simulink model "Motoring_Gear"  (R2024a)
settings: Solver=VariableStepAuto  StartTime=0.0  StopTime=2  FixedStep=1e-6  MaxStep=1e-6  RelTol=1e-6
values from neighbouring files (symbols this model uses):
  B_mod = 0    [Motoring_Gear_param.m]
  Bdc = 1e-4    (= 0.0001)    [Motoring_Gear_param.m]
  BL = 5    [Motoring_Gear_param.m]
  Bs = 1e10    (= 10000000000)    [Motoring_Gear_param.m]
  Bsn = 0    [Motoring_Gear_param.m]
  flux = 0.0563    [Motoring_Gear_param.m]
  J_mod = 5.71e-4    (= 0.000571)    [Motoring_Gear_param.m]
  Jdc = 0.0003    [Motoring_Gear_param.m]
  Jsn = 3.16e-4    (= 0.000316)    [Motoring_Gear_param.m]
  Kag = 0.001    [Motoring_Gear_param.m]
  Kc = 1000000    [Motoring_Gear_param.m]
  Ke = 0.0164    [Motoring_Gear_param.m]
  Kt = 0.0164    [Motoring_Gear_param.m]
  Ld = 3e-5    (= 3e-05)    [Motoring_Gear_param.m]
  Ldc = 8.76e-5    (= 8.76e-05)    [Motoring_Gear_param.m]
  Lq = 3e-5    (= 3e-05)    [Motoring_Gear_param.m]
  Pa = 2    [Motoring_Gear_param.m]
  Psn = 9    [Motoring_Gear_param.m]
  q_mod = 11    [Motoring_Gear_param.m]
  Rs = 0.01    [Motoring_Gear_param.m]
  Rs_dc = 0.01    [Motoring_Gear_param.m]
  velocity_Ki_pi = Bdc*motor_bw    (= 0.0628318530718)    [Motoring_Gear_param.m]
  velocity_Kp_pi = Jdc*motor_bw    (= 0.188495559215)    [Motoring_Gear_param.m]
libraries: cstblocks x2
(part 2 of 2)

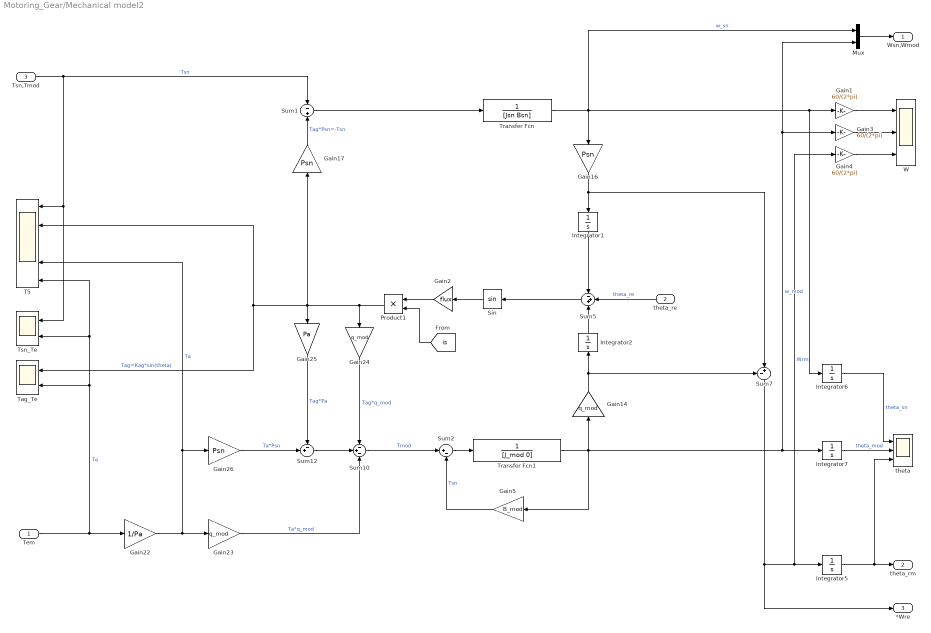
== system Motoring_Gear/Mechanical model2 ==
  Tem : Inport
  theta_re : Inport  Port=2
  Tsn,Tmod : Inport  Port=3
  Gain1 : Gain  Gain=60/(2*pi)
  Gain14 : Gain  Gain=q_mod
  Gain16 : Gain  Gain=Psn
  Gain17 : Gain  Gain=Psn
  Gain2 : Gain  Gain=flux
  Gain22 : Gain  Gain=1/Pa
  Gain23 : Gain  Gain=q_mod
  Gain24 : Gain  Gain=q_mod
  Gain25 : Gain  Gain=Pa
  Gain26 : Gain  Gain=Psn
  Gain3 : Gain  Gain=60/(2*pi)
  Gain4 : Gain  Gain=60/(2*pi)
  Gain5 : Gain  Gain=B_mod
  Integrator{1..2,5..7} (5 alike) : Integrator
  Mux : Mux  Inputs=2
  Product1 : Product
  Sin : Trigonometry
  Sum1 : Sum  Inputs=-|+
  Sum10 : Sum  Inputs=-+-
  Sum12 : Sum  Inputs=-+|
  Sum2 : Sum  Inputs=|+-
  Sum5 : Sum  Inputs=-++
  Sum7 : Sum  Inputs=-+|
  T5 : Scope  NumInputPorts=5
  Tag_Te : Scope  NumInputPorts=2
  Transfer Fcn : TransferFcn  Denominator=[Jsn Bsn]
  Transfer Fcn1 : TransferFcn  Denominator=[J_mod 0]
  Tsn_Te : Scope  NumInputPorts=2
  W : Scope  NumInputPorts=3
  theta : Scope  NumInputPorts=3
  Wsn,Wmod : Outport
  theta_rm : Outport  Port=2
  *Wre : Outport  Port=3
  wires:
  Gain4/1 -> W/3
  Gain3/1 -> W/2
  Gain1/1 -> W/1
  Tsn,Tmod/1 -> Sum1/1, Tsn_Te/1, T5/1  "Tsn"
  Mux/1 -> Wsn,Wmod/1
  Transfer Fcn/1 -> Mux/1, Gain16/1, Integrator6/1, Gain1/1  "w_sn"
  Gain17/1 -> Sum1/2  "Tag*Psn=-Tsn"
  Gain16/1 -> Integrator1/1, Sum7/2
  Product1/1 -> Gain25/1, T5/2, Tag_Te/1, Gain17/1, Gain24/1  "Tag=Kag*sin(theta)"
  Sum5/1 -> Sin/1
  Transfer Fcn1/1 -> Gain14/1, Gain3/1, Mux/2, Integrator7/1, Gain5/1  "w_mod"
  Tem/1 -> Gain22/1, T5/5, Tsn_Te/2, Tag_Te/2  "Te"
  Sum7/1 -> *Wre/1, Gain4/1, Integrator5/1  "Wrm"
  Gain25/1 -> Sum12/1  "Tag*Pa"
  Gain22/1 -> Gain26/1, T5/4, Gain23/1  "Ta"
  Gain26/1 -> Sum12/2  "Ta*Psn"
  Sum12/1 -> Sum10/2
  Gain24/1 -> Sum10/1  "Tag*q_mod"
  Gain23/1 -> Sum10/3  "Ta*q_mod"
  Sum10/1 -> Sum2/1  "Tmod"
  Integrator5/1 -> theta_rm/1, theta/3
  Integrator6/1 -> theta/1  "theta_sn"
  Integrator7/1 -> theta/2  "theta_mod"
  Sum1/1 -> Transfer Fcn/1
  theta_re/1 -> Sum5/2  "theta_re"
  Sum2/1 -> Transfer Fcn1/1
  Integrator1/1 -> Sum5/1
  Integrator2/1 -> Sum5/3
  Gain14/1 -> Integrator2/1, Sum7/1
  Gain5/1 -> Sum2/2  "Tsn"
  [is] -> Product1/2
  Gain2/1 -> Product1/1
  Sin/1 -> Gain2/1

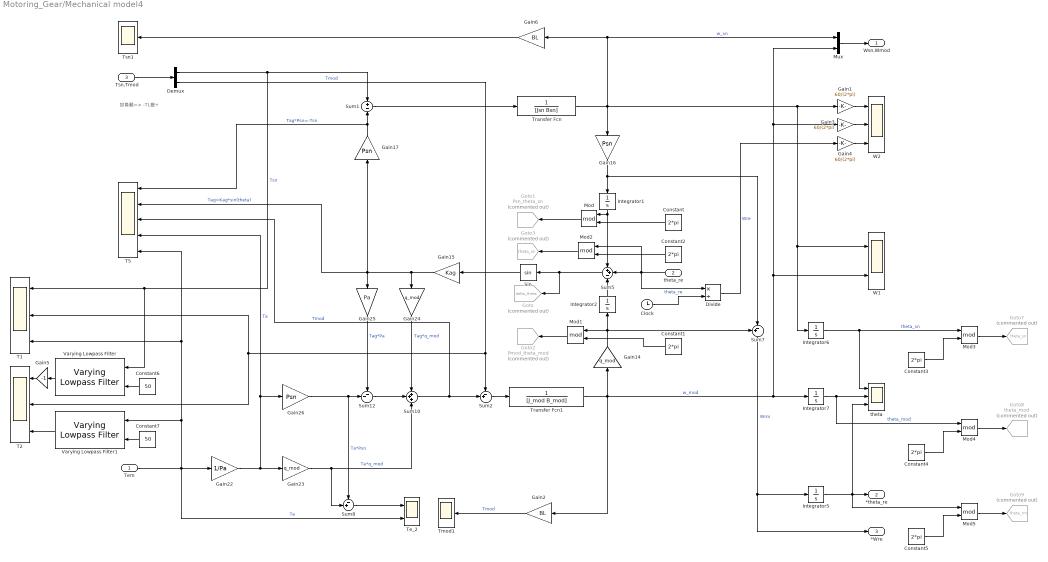
== system Motoring_Gear/Mechanical model4 ==
  note: 加負載=> -TL變+
  Tem : Inport
  theta_re : Inport  Port=2
  Tsn,Tmod : Inport  Port=3
  Clock : Clock
  Constant{,1..5} (6 alike) : Constant  Value=2*pi
  Constant6 : Constant  Value=50
  Constant7 : Constant  Value=50
  Demux : Demux  Outputs=2
  Divide : Product  Inputs=*/
  Gain1 : Gain  Gain=60/(2*pi)
  Gain14 : Gain  Gain=q_mod
  Gain15 : Gain  Gain=Kag
  Gain16 : Gain  Gain=Psn
  Gain17 : Gain  Gain=Psn
  Gain2 : Gain  Gain=BL
  Gain22 : Gain  Gain=1/Pa
  Gain23 : Gain  Gain=q_mod
  Gain24 : Gain  Gain=q_mod
  Gain25 : Gain  Gain=Pa
  Gain26 : Gain  Gain=Psn
  Gain3 : Gain  Gain=60/(2*pi)
  Gain4 : Gain  Gain=60/(2*pi)
  Gain5 : Gain  Gain=-1
  Gain6 : Gain  Gain=BL
  Goto : Goto  Commented=on  GotoTag=delta_theta  TagVisibility=global
  Goto1 : Goto  Commented=on  GotoTag=Psn_theta_sn  TagVisibility=global
  Goto2 : Goto  Commented=on  GotoTag=Pmod_theta_mod  TagVisibility=global
  Goto3 : Goto  Commented=on  GotoTag=theta_re  TagVisibility=global
  Goto7 : Goto  Commented=on  GotoTag=theta_sn  TagVisibility=global
  Goto8 : Goto  Commented=on  GotoTag=theta_mod  TagVisibility=global
  Goto9 : Goto  Commented=on  GotoTag=theta_rm  TagVisibility=global
  Integrator{1..2,5..7} (5 alike) : Integrator
  Mod{,1..5} (6 alike) : Math  Operator=mod
  Mux : Mux  Inputs=2
  Sin : Trigonometry
  Sum1 : Sum  Inputs=+|-
  Sum10 : Sum  Inputs=+++
  Sum12 : Sum  Inputs=--|
  Sum2 : Sum  Inputs=-+|
  Sum5 : Sum  Inputs=++-
  Sum7 : Sum  Inputs=+-|
  Sum8 : Sum  Inputs=-+|
  T1 : Scope  NumInputPorts=3
  T2 : Scope  NumInputPorts=3
  T5 : Scope  NumInputPorts=5
  Te_2 : Scope  NumInputPorts=2
  Tmod1 : Scope
  Transfer Fcn : TransferFcn  Denominator=[Jsn Bsn]
  Transfer Fcn1 : TransferFcn  Denominator=[J_mod B_mod]
  Tsn1 : Scope
  Varying Lowpass Filter : cstblocks/Linear Parameter Varying/Varying Lowpass Filter  N=1
  Varying Lowpass Filter1 : cstblocks/Linear Parameter Varying/Varying Lowpass Filter  N=1
  W1 : Scope  NumInputPorts=2
  W2 : Scope  NumInputPorts=3
  theta : Scope  NumInputPorts=3
  Wsn,Wmod : Outport
  *theta_re : Outport  Port=2
  *Wre : Outport  Port=3
  wires:
  Mod5/1 -> Goto9/1
  Constant5/1 -> Mod5/2
  Constant4/1 -> Mod4/2
  Mod4/1 -> Goto8/1
  Mod3/1 -> Goto7/1
  Constant3/1 -> Mod3/2
  Constant2/1 -> Mod2/2
  Mod2/1 -> Goto3/1
  Constant1/1 -> Mod1/2
  Gain14/1 -> Sum7/1, Mod1/1, Integrator2/1
  Mod1/1 -> Goto2/1
  Mod/1 -> Goto1/1
  Constant/1 -> Mod/2
  Integrator2/1 -> Sum5/3
  Integrator1/1 -> Mod/1, Sum5/1
  Sum2/1 -> Transfer Fcn1/1
  theta_re/1 -> Mod2/1, Divide/1, Sum5/2  "theta_re"
  Sum1/1 -> Transfer Fcn/1
  Sin/1 -> Gain15/1
  Integrator7/1 -> Mod4/1, theta/2  "theta_mod"
  Integrator6/1 -> Mod3/1, theta/1  "theta_sn"
  Integrator5/1 -> theta/3, *theta_re/1, Mod5/1
  Sum10/1 -> Sum2/2, T5/3  "Tmod"
  Gain23/1 -> Sum10/3, Sum8/2  "Ta*q_mod"
  Gain24/1 -> Sum10/1  "Tag*q_mod"
  Sum12/1 -> Sum10/2
  Gain26/1 -> Sum12/2, Sum8/1  "Ta*Psn"
  Gain22/1 -> Gain23/1, T5/4, Gain26/1  "Ta"
  Gain25/1 -> Sum12/1  "Tag*Pa"
  Sum7/1 -> Integrator5/1, *Wre/1  "Wrm"
  Tem/1 -> Te_2/2, Varying Lowpass Filter1/1, T1/3, T5/5, Gain22/1  "Te"
  Transfer Fcn1/1 -> Gain2/1, Integrator7/1, W1/2, Gain3/1, Mux/2, Gain14/1  "w_mod"
  Sum5/1 -> Sin/1, Goto/1
  Gain15/1 -> Gain24/1, Gain17/1, T5/2, Gain25/1  "Tag=Kag*sin(theta)"
  Gain16/1 -> Sum7/2, Integrator1/1
  Gain17/1 -> Sum1/2, T5/1  "Tag*Psn=-Tsn"
  Transfer Fcn/1 -> Gain1/1, W1/1, Integrator6/1, Gain16/1, Mux/1, Gain6/1  "w_sn"
  Sum8/1 -> Te_2/1
  Gain6/1 -> Tsn1/1
  Gain2/1 -> Tmod1/1  "Tmod"
  Mux/1 -> Wsn,Wmod/1
  Tsn,Tmod/1 -> Demux/1
  Demux/1 -> Varying Lowpass Filter/1, T1/1, Sum1/1  "Tsn"
  Demux/2 -> Sum2/1, T1/2, T2/2  "Tmod"
  Gain1/1 -> W2/1
  Gain3/1 -> W2/2
  Gain4/1 -> W2/3
  Clock/1 -> Divide/2
  Divide/1 -> Gain4/1  "Wre"
  Constant6/1 -> Varying Lowpass Filter/2
  Varying Lowpass Filter1/1 -> T2/3
  Constant7/1 -> Varying Lowpass Filter1/2
  Gain5/1 -> T2/1
  Varying Lowpass Filter/1 -> Gain5/1

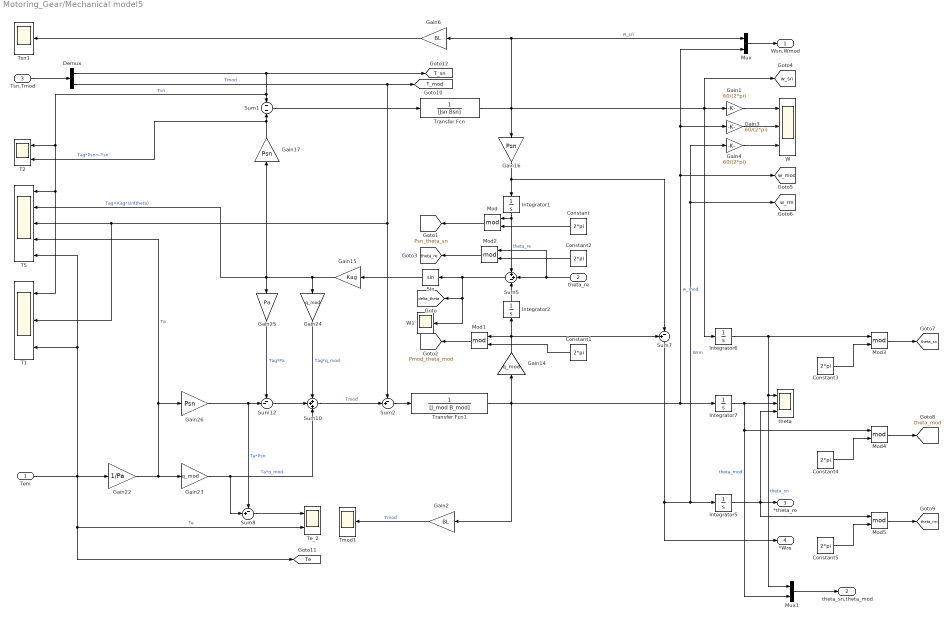
== system Motoring_Gear/Mechanical model5 ==
  Tem : Inport
  theta_re : Inport  Port=2
  Tsn,Tmod : Inport  Port=3
  Constant{,1..5} (6 alike) : Constant  Value=2*pi
  Demux : Demux  Outputs=2
  Gain1 : Gain  Gain=60/(2*pi)
  Gain14 : Gain  Gain=q_mod
  Gain15 : Gain  Gain=Kag
  Gain16 : Gain  Gain=Psn
  Gain17 : Gain  Gain=Psn
  Gain2 : Gain  Gain=BL
  Gain22 : Gain  Gain=1/Pa
  Gain23 : Gain  Gain=q_mod
  Gain24 : Gain  Gain=q_mod
  Gain25 : Gain  Gain=Pa
  Gain26 : Gain  Gain=Psn
  Gain3 : Gain  Gain=60/(2*pi)
  Gain4 : Gain  Gain=60/(2*pi)
  Gain6 : Gain  Gain=BL
  Integrator{1..2,5..7} (5 alike) : Integrator
  Mod{,1..5} (6 alike) : Math  Operator=mod
  Mux : Mux  Inputs=2
  Mux1 : Mux  Inputs=2
  Sin : Trigonometry
  Sum1 : Sum  Inputs=-|-
  Sum10 : Sum  Inputs=+++
  Sum12 : Sum  Inputs=--|
  Sum2 : Sum  Inputs=-+|
  Sum5 : Sum  Inputs=++-
  Sum7 : Sum  Inputs=+-|
  Sum8 : Sum  Inputs=-+|
  T1 : Scope  NumInputPorts=3
  T2 : Scope  NumInputPorts=2
  T5 : Scope  NumInputPorts=5
  Te_2 : Scope  NumInputPorts=2
  Tmod1 : Scope
  Transfer Fcn : TransferFcn  Denominator=[Jsn Bsn]
  Transfer Fcn1 : TransferFcn  Denominator=[J_mod B_mod]
  Tsn1 : Scope
  W : Scope  NumInputPorts=3
  W1 : Scope
  theta : Scope  NumInputPorts=3
  Wsn,Wmod : Outport
  theta_sn,theta_mod : Outport  Port=2
  *theta_re : Outport  Port=3
  *Wre : Outport  Port=4
  tag scope: Pmod_theta_mod=global, Psn_theta_sn=global, T_mod=global, T_sn=global, Te=global, delta_theta=global, theta_mod=global, theta_re=global, theta_rm=global, theta_sn=global, w_mod=global, w_rm=global, w_sn=global
  wires:
  Mux1/1 -> theta_sn,theta_mod/1
  Mod5/1 -> [theta_rm]
  Constant5/1 -> Mod5/2
  Constant4/1 -> Mod4/2
  Mod4/1 -> [theta_mod]
  Mod3/1 -> [theta_sn]
  Constant3/1 -> Mod3/2
  Constant2/1 -> Mod2/2
  Mod2/1 -> [theta_re]
  Constant1/1 -> Mod1/2
  Gain14/1 -> Sum7/1, Mod1/1, Integrator2/1
  Mod1/1 -> [Pmod_theta_mod]
  Mod/1 -> [Psn_theta_sn]
  Constant/1 -> Mod/2
  Integrator2/1 -> Sum5/3
  Integrator1/1 -> Mod/1, Sum5/1
  Sum2/1 -> Transfer Fcn1/1
  theta_re/1 -> Sum5/2, Mod2/1  "theta_re"
  Sum1/1 -> Transfer Fcn/1
  Sin/1 -> Gain15/1
  Integrator7/1 -> Mod4/1, Mux1/2, theta/2  "theta_mod"
  Integrator6/1 -> Mod3/1, Mux1/1, theta/1  "theta_sn"
  Integrator5/1 -> theta/3, *theta_re/1, Mod5/1
  Sum10/1 -> Sum2/2  "Tmod"
  Gain23/1 -> Sum10/3, Sum8/2  "Ta*q_mod"
  Gain24/1 -> Sum10/1  "Tag*q_mod"
  Sum12/1 -> Sum10/2
  Gain26/1 -> Sum12/2, Sum8/1  "Ta*Psn"
  Gain22/1 -> Gain23/1, T5/4, Gain26/1  "Ta"
  Gain25/1 -> Sum12/1  "Tag*Pa"
  Sum7/1 -> Integrator5/1, Gain4/1, [w_rm], *Wre/1  "Wrm"
  Tem/1 -> Te_2/2, [Te], T5/5, T1/3, Gain22/1  "Te"
  Transfer Fcn1/1 -> Gain2/1, Integrator7/1, Mux/2, Gain3/1, [w_mod], Gain14/1  "w_mod"
  Sum5/1 -> Sin/1, W1/1, [delta_theta]
  Gain15/1 -> Gain24/1, Gain17/1, T5/2, Gain25/1  "Tag=Kag*sin(theta)"
  Gain16/1 -> Sum7/2, Integrator1/1
  Gain17/1 -> T2/2, Sum1/2  "Tag*Psn=-Tsn"
  Transfer Fcn/1 -> Gain1/1, [w_sn], Integrator6/1, Gain16/1, Mux/1, Gain6/1  "w_sn"
  Sum8/1 -> Te_2/1
  Gain6/1 -> Tsn1/1
  Gain2/1 -> Tmod1/1  "Tmod"
  Mux/1 -> Wsn,Wmod/1
  Tsn,Tmod/1 -> Demux/1
  Demux/1 -> [T_sn], T2/1, T1/1, T5/1, Sum1/1  "Tsn"
  Demux/2 -> [T_mod], Sum2/1, T1/2, T5/3  "Tmod"
  Gain1/1 -> W/1
  Gain3/1 -> W/2
  Gain4/1 -> W/3

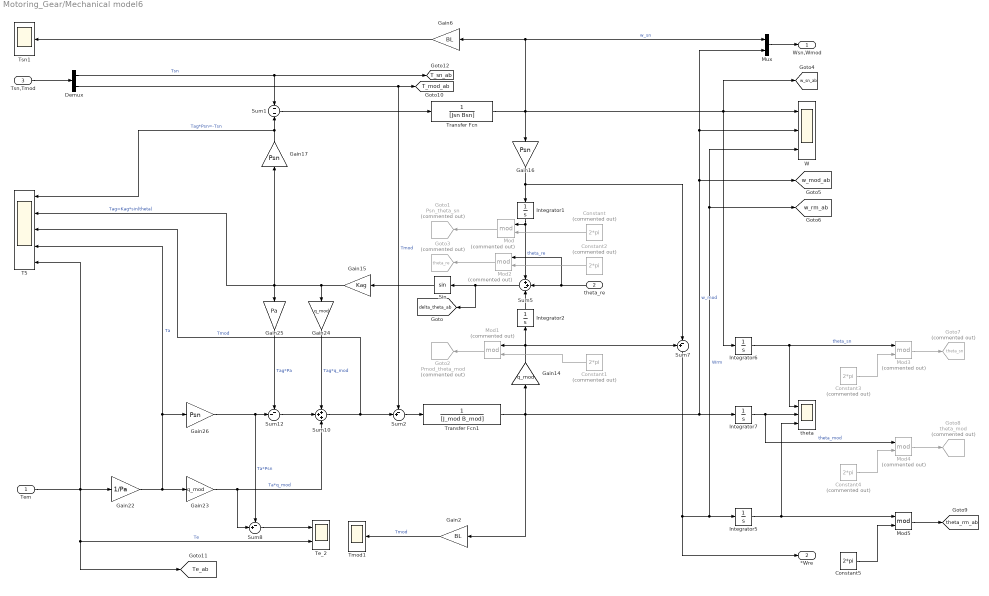
== system Motoring_Gear/Mechanical model6 ==
  Tem : Inport
  theta_re : Inport  Port=2
  Tsn,Tmod : Inport  Port=3
  Constant{,1..4} (5 alike) : Constant  Commented=on  Value=2*pi
  Constant5 : Constant  Value=2*pi
  Demux : Demux  Outputs=2
  Gain14 : Gain  Gain=q_mod
  Gain15 : Gain  Gain=Kag
  Gain16 : Gain  Gain=Psn
  Gain17 : Gain  Gain=Psn
  Gain2 : Gain  Gain=BL
  Gain22 : Gain  Gain=1/Pa
  Gain23 : Gain  Gain=q_mod
  Gain24 : Gain  Gain=q_mod
  Gain25 : Gain  Gain=Pa
  Gain26 : Gain  Gain=Psn
  Gain6 : Gain  Gain=BL
  Goto1 : Goto  Commented=on  GotoTag=Psn_theta_sn  TagVisibility=global
  Goto2 : Goto  Commented=on  GotoTag=Pmod_theta_mod  TagVisibility=global
  Goto3 : Goto  Commented=on  GotoTag=theta_re  TagVisibility=global
  Goto7 : Goto  Commented=on  GotoTag=theta_sn  TagVisibility=global
  Goto8 : Goto  Commented=on  GotoTag=theta_mod  TagVisibility=global
  Integrator{1..2,5..7} (5 alike) : Integrator
  Mod{,1..4} (5 alike) : Math  Commented=on  Operator=mod
  Mod5 : Math  Operator=mod
  Mux : Mux  Inputs=2
  Sin : Trigonometry
  Sum1 : Sum  Inputs=-|-
  Sum10 : Sum  Inputs=+++
  Sum12 : Sum  Inputs=--|
  Sum2 : Sum  Inputs=-+|
  Sum5 : Sum  Inputs=++-
  Sum7 : Sum  Inputs=+-|
  Sum8 : Sum  Inputs=-+|
  T5 : Scope  NumInputPorts=5
  Te_2 : Scope  NumInputPorts=2
  Tmod1 : Scope
  Transfer Fcn : TransferFcn  Denominator=[Jsn Bsn]
  Transfer Fcn1 : TransferFcn  Denominator=[J_mod B_mod]
  Tsn1 : Scope
  W : Scope  NumInputPorts=3
  theta : Scope  NumInputPorts=3
  Wsn,Wmod : Outport
  *Wre : Outport  Port=2
  tag scope: T_mod_ab=global, T_sn_ab=global, Te_ab=global, delta_theta_ab=global, theta_rm_ab=global, w_mod_ab=global, w_rm_ab=global, w_sn_ab=global
  wires:
  Demux/2 -> [T_mod_ab], Sum2/1  "Tmod"
  Demux/1 -> [T_sn_ab], Sum1/1  "Tsn"
  Tsn,Tmod/1 -> Demux/1
  Mux/1 -> Wsn,Wmod/1
  Gain2/1 -> Tmod1/1  "Tmod"
  Gain6/1 -> Tsn1/1
  Sum8/1 -> Te_2/1
  Transfer Fcn/1 -> Gain6/1, Mux/1, Gain16/1, Integrator6/1, [w_sn_ab], W/1  "w_sn"
  Gain17/1 -> T5/1, Sum1/2  "Tag*Psn=-Tsn"
  Gain16/1 -> Integrator1/1, Sum7/2
  Gain15/1 -> Gain25/1, T5/2, Gain17/1, Gain24/1  "Tag=Kag*sin(theta)"
  Sum5/1 -> [delta_theta_ab], Sin/1
  Transfer Fcn1/1 -> Gain14/1, [w_mod_ab], W/2, Mux/2, Integrator7/1, Gain2/1  "w_mod"
  Tem/1 -> Gain22/1, T5/5, [Te_ab], Te_2/2  "Te"
  Sum7/1 -> *Wre/1, [w_rm_ab], W/3, Integrator5/1  "Wrm"
  Gain25/1 -> Sum12/1  "Tag*Pa"
  Gain22/1 -> Gain26/1, T5/4, Gain23/1  "Ta"
  Gain26/1 -> Sum8/1, Sum12/2  "Ta*Psn"
  Sum12/1 -> Sum10/2
  Gain24/1 -> Sum10/1  "Tag*q_mod"
  Gain23/1 -> Sum8/2, Sum10/3  "Ta*q_mod"
  Sum10/1 -> T5/3, Sum2/2  "Tmod"
  Integrator5/1 -> Mod5/1, theta/3
  Integrator6/1 -> theta/1, Mod3/1  "theta_sn"
  Integrator7/1 -> theta/2, Mod4/1  "theta_mod"
  Sin/1 -> Gain15/1
  Sum1/1 -> Transfer Fcn/1
  theta_re/1 -> Mod2/1, Sum5/2  "theta_re"
  Sum2/1 -> Transfer Fcn1/1
  Integrator1/1 -> Sum5/1, Mod/1
  Integrator2/1 -> Sum5/3
  Constant/1 -> Mod/2
  Mod/1 -> Goto1/1
  Mod1/1 -> Goto2/1
  Gain14/1 -> Integrator2/1, Mod1/1, Sum7/1
  Constant1/1 -> Mod1/2
  Mod2/1 -> Goto3/1
  Constant2/1 -> Mod2/2
  Constant3/1 -> Mod3/2
  Mod3/1 -> Goto7/1
  Mod4/1 -> Goto8/1
  Constant4/1 -> Mod4/2
  Constant5/1 -> Mod5/2
  Mod5/1 -> [theta_rm_ab]

== system Motoring_Gear/Speed Estimator2 ==
  theta_re_res : Inport
  Clock : Clock
  Divide : Product  Inputs=/*
  w_re_res : Scope
  w_re_res1 : Outport
  tag scope: w_rm_res=global
  wires:
  theta_re_res/1 -> Divide/2
  Divide/1 -> w_re_res1/1, [w_rm_res], w_re_res/1
  Clock/1 -> Divide/1

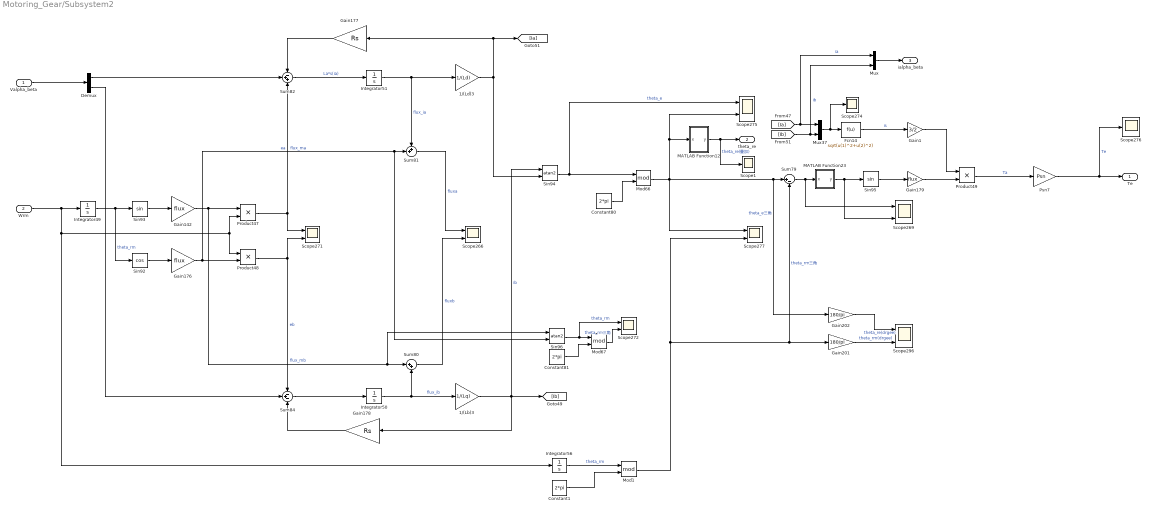
== system Motoring_Gear/Subsystem2 ==
  Valpha_beta : Inport
  Wrm : Inport  Port=2
  1/(Lb)3 : Gain  Gain=1/(Lq)
  1/(Ld)3 : Gain  Gain=1/(Ld)
  Constant1 : Constant  Value=2*pi
  Constant80 : Constant  Value=2*pi
  Constant81 : Constant  Value=2*pi
  Demux : Demux  Outputs=2
  Fcn14 : Fcn  Expr=sqrt(u(1)^2+u(2)^2)
  Gain1 : Gain  Gain=3/2
  Gain142 : Gain  Gain=flux
  Gain176 : Gain  Gain=flux
  Gain177 : Gain  Gain=Rs
  Gain178 : Gain  Gain=Rs
  Gain179 : Gain  Gain=flux
  Gain201 : Gain  Gain=180/pi
  Gain202 : Gain  Gain=180/pi
  Integrator{49..51,56} (4 alike) : Integrator
  MATLAB Function12 : MATLAB Function  TreatAsAtomicUnit=on
  MATLAB Function23 : MATLAB Function  TreatAsAtomicUnit=on
  Mod1 : Math  Operator=mod  OutputSignalType=real
  Mod66 : Math  Operator=mod  OutputSignalType=real
  Mod67 : Math  Operator=mod  OutputSignalType=real
  Mux : Mux  Inputs=2
  Mux37 : Mux  Inputs=2
  Product47 : Product
  Product48 : Product
  Product49 : Product
  Psn7 : Gain  Gain=Psn
  Scope1 : Scope
  Scope{266,269,271..272,275,277,296} (7 alike) : Scope  NumInputPorts=2
  Scope274 : Scope
  Scope276 : Scope
  Sin92 : Trigonometry  Operator=cos
  Sin93 : Trigonometry
  Sin94 : Trigonometry  Operator=atan2
  Sin95 : Trigonometry
  Sin96 : Trigonometry  Operator=atan2
  Sum79 : Sum  Inputs=|+-
  Sum80 : Sum  Inputs=|++
  Sum81 : Sum  Inputs=++|
  Sum82 : Sum  Inputs=-++
  Sum84 : Sum  Inputs=-+-
  Te : Outport
  theta_re : Outport  Port=2
  ialpha_beta : Outport  Port=3
  wires:
  Constant1/1 -> Mod1/2
  Integrator56/1 -> Mod1/1  "theta_rm"
  MATLAB Function12/1(y) -> theta_re/1, Scope1/1  "theta_re(疊加)"
  Sum82/1 -> Integrator51/1  "La*s(ia)"
  1/(Lb)3/1 -> Gain178/1, Sin94/1, [Ib]  "ib"
  Fcn14/1 -> Gain1/1  "is"
  MATLAB Function23/1(y) -> Scope269/2, Sin95/1
  Mod67/1 -> Scope272/2  "theta_rm三角"
  Mod1/1 -> Gain201/1, Sum79/2, Scope277/2  "theta_rm三角"
  Integrator51/1 -> 1/(Ld)3/1, Sum81/1  "flux_ia"
  Gain201/1 -> Scope296/2  "theta_rm(drgee)"
  Psn7/1 -> Te/1, Scope276/1  "Te"
  Mod66/1 -> Gain202/1, Sum79/1, Scope277/1, Scope275/2, MATLAB Function12/1(x)  "theta_e三角"
  Product48/1 -> Sum84/1, Scope271/2  "eb"
  Product49/1 -> Psn7/1  "Ta"
  Sin94/1 -> Mod66/1, Scope275/1  "theta_e"
  Gain142/1 -> Product47/1, Sum80/1, Sin96/1  "flux_mb"
  Gain176/1 -> Product48/2, Sum81/2, Sin96/2  "flux_ma"
  Sum80/1 -> Scope266/2  "fluxb"
  Gain1/1 -> Product49/1
  Sin93/1 -> Gain142/1
  Constant81/1 -> Mod67/2
  Mux37/1 -> Fcn14/1, Scope274/1
  Integrator49/1 -> Sin93/1, Sin92/1  "theta_rm"
  1/(Ld)3/1 -> [Ia], Gain177/1, Sin94/2
  Sin96/1 -> Mod67/1, Scope272/1  "theta_rm"
  Integrator50/1 -> Sum80/2, 1/(Lb)3/1  "flux_ib"
  Sum84/1 -> Integrator50/1
  Gain179/1 -> Product49/2
  Gain202/1 -> Scope296/1  "theta_re(drgee)"
  Sum79/1 -> Scope269/1, MATLAB Function23/1(x)
  Sum81/1 -> Scope266/1  "fluxa"
  Sin92/1 -> Gain176/1
  Gain178/1 -> Sum84/3
  Constant80/1 -> Mod66/2
  [Ib] -> Mux/2, Mux37/2  "ib"
  Sin95/1 -> Gain179/1
  [Ia] -> Mux/1, Mux37/1  "ia"
  Product47/1 -> Sum82/3, Scope271/1  "ea"
  Gain177/1 -> Sum82/1
  Wrm/1 -> Product47/2, Product48/1, Integrator56/1, Integrator49/1
  Demux/1 -> Sum82/2
  Valpha_beta/1 -> Demux/1
  Demux/2 -> Sum84/2
  Mux/1 -> ialpha_beta/1

== system Motoring_Gear/Subsystem6 ==
  Te : Inport
  TL : Inport  Port=2
  Gain5 : Gain  Gain=Psn
  Integrator7 : Integrator
  Sum1 : Sum  Inputs=-+|
  T : Scope
  Transfer Fcn1 : TransferFcn  Denominator=[Jsn Bsn]
  W : Scope  NumInputPorts=2
  t_rm : Scope
  wsn : Outport
  theta_rm : Outport  Port=2
  Wrm : Outport  Port=3
  wires:
  TL/1 -> Sum1/1
  Te/1 -> T/1, Sum1/2
  Transfer Fcn1/1 -> wsn/1, W/1, Gain5/1  "Wsn"
  Sum1/1 -> Transfer Fcn1/1
  Gain5/1 -> Integrator7/1, Wrm/1, W/2  "Wrm"
  Integrator7/1 -> theta_rm/1, t_rm/1

== system Motoring_Gear/abc//alpha-beta1 ==
  vabc : Inport
  ialpha_beta : Inport  Port=2
  Subsystem1 : Subsystem
  Subsystem3 : Subsystem
      settings: PortSchema="{\"entries\":[{\"content\":{\"sides\":[{\"content\":{\"connectorIds\":[\"Out1\"]},\"type\":\"ConnectorPlacement.EquallySpacedRectSide\",\"uuid\":\"b8dbbc21-c1f4-4ee6-a4ae-0919678ef684\"},{\"content\":{\"connectorIds\":[\"In1\"],\"side\":\"RIGHT\"},\"type\":\"ConnectorPlacement.EquallySpacedRectSide\",\"uuid\":\"61e1bbf5-e287-4b89-b804-9623b46ea559\"},{\"content\":{\"connectorIds\":[],\"side\":\"TOP\"},\"type\":\"ConnectorPlacement.EquallySpacedRectSide\",\"uuid\":\"efb7ccb4-1c85-4d0f-b3e5-0bebc17d0910\"}]},\"type\":\"ConnectorPlacement.EquallySpacedConnector\",\"uuid\":\"801d87a2-54d2-4006-a4d4-92ff44eea017\"}],\"packageUris\":[\"http://schema.mathworks.com/mf0/Connector/R2020b\"],\"version\":\"1.0\"}"
  valpha_beta : Outport
  iabc : Outport  Port=2
  wires:
  Subsystem3/1(iabc) -> iabc/1
  Subsystem1/1(valpha_beta1) -> valpha_beta/1
  ialpha_beta/1 -> Subsystem3/1(ialpha_beta)
  vabc/1 -> Subsystem1/1(vabc1)

== system Motoring_Gear/abc//alpha-beta3 ==
  vabc : Inport
  ialpha_beta : Inport  Port=2
  Subsystem1 : Subsystem
  Subsystem3 : Subsystem
      settings: PortSchema="{\"entries\":[{\"content\":{\"sides\":[{\"content\":{\"connectorIds\":[\"Out1\"]},\"type\":\"ConnectorPlacement.EquallySpacedRectSide\",\"uuid\":\"b8dbbc21-c1f4-4ee6-a4ae-0919678ef684\"},{\"content\":{\"connectorIds\":[\"In1\"],\"side\":\"RIGHT\"},\"type\":\"ConnectorPlacement.EquallySpacedRectSide\",\"uuid\":\"61e1bbf5-e287-4b89-b804-9623b46ea559\"},{\"content\":{\"connectorIds\":[],\"side\":\"TOP\"},\"type\":\"ConnectorPlacement.EquallySpacedRectSide\",\"uuid\":\"efb7ccb4-1c85-4d0f-b3e5-0bebc17d0910\"}]},\"type\":\"ConnectorPlacement.EquallySpacedConnector\",\"uuid\":\"801d87a2-54d2-4006-a4d4-92ff44eea017\"}],\"packageUris\":[\"http://schema.mathworks.com/mf0/Connector/R2020b\"],\"version\":\"1.0\"}"
  valpha_beta : Outport
  iabc : Outport  Port=2
  wires:
  vabc/1 -> Subsystem1/1(vabc1)
  ialpha_beta/1 -> Subsystem3/1(ialpha_beta)
  Subsystem1/1(valpha_beta1) -> valpha_beta/1
  Subsystem3/1(iabc) -> iabc/1

== system Motoring_Gear/abc//alpha-beta4 ==
  vabc : Inport
  ialpha_beta : Inport  Port=2
  Subsystem1 : Subsystem
  Subsystem3 : Subsystem
      settings: PortSchema="{\"entries\":[{\"content\":{\"sides\":[{\"content\":{\"connectorIds\":[\"Out1\"]},\"type\":\"ConnectorPlacement.EquallySpacedRectSide\",\"uuid\":\"b8dbbc21-c1f4-4ee6-a4ae-0919678ef684\"},{\"content\":{\"connectorIds\":[\"In1\"],\"side\":\"RIGHT\"},\"type\":\"ConnectorPlacement.EquallySpacedRectSide\",\"uuid\":\"61e1bbf5-e287-4b89-b804-9623b46ea559\"},{\"content\":{\"connectorIds\":[],\"side\":\"TOP\"},\"type\":\"ConnectorPlacement.EquallySpacedRectSide\",\"uuid\":\"efb7ccb4-1c85-4d0f-b3e5-0bebc17d0910\"}]},\"type\":\"ConnectorPlacement.EquallySpacedConnector\",\"uuid\":\"801d87a2-54d2-4006-a4d4-92ff44eea017\"}],\"packageUris\":[\"http://schema.mathworks.com/mf0/Connector/R2020b\"],\"version\":\"1.0\"}"
  valpha_beta : Outport
  iabc : Outport  Port=2
  wires:
  vabc/1 -> Subsystem1/1(vabc1)
  ialpha_beta/1 -> Subsystem3/1(ialpha_beta)
  Subsystem1/1(valpha_beta1) -> valpha_beta/1
  Subsystem3/1(iabc) -> iabc/1

== system Motoring_Gear/alpha-beta//dq1 ==
  valpha_beta : Inport
  *theta_re : Inport  Port=2
  idqs : Inport  Port=3
  Demux : Demux  Outputs=2
  Demux1 : Demux  Outputs=2
  Subsystem : Subsystem
  Subsystem1 : Subsystem
  vdqs : Outport
  ialpha_beta : Outport  Port=2
  wires:
  Subsystem/1(vdqs) -> vdqs/1
  Demux/2 -> Subsystem/2(vbeta)
  Demux1/2 -> Subsystem1/2(iq)
  Demux/1 -> Subsystem/1(valpha)
  Demux1/1 -> Subsystem1/1(id)
  *theta_re/1 -> Subsystem/3(*theta_re), Subsystem1/3(*theta_re1)
  valpha_beta/1 -> Demux/1
  idqs/1 -> Demux1/1
  Subsystem1/1(ialpha_beta) -> ialpha_beta/1

== system Motoring_Gear/alpha-beta//dq2 ==
  valpha_beta : Inport
  *theta_re : Inport  Port=2
  idqs : Inport  Port=3
  Demux : Demux  Outputs=2
  Demux1 : Demux  Outputs=2
  Subsystem : Subsystem
  Subsystem1 : Subsystem
  vdqs : Outport
  ialpha_beta : Outport  Port=2
  wires:
  Subsystem1/1(ialpha_beta) -> ialpha_beta/1
  idqs/1 -> Demux1/1
  valpha_beta/1 -> Demux/1
  *theta_re/1 -> Subsystem1/3(*theta_re1), Subsystem/3(*theta_re)
  Demux1/1 -> Subsystem1/1(id)
  Demux/1 -> Subsystem/1(valpha)
  Demux1/2 -> Subsystem1/2(iq)
  Demux/2 -> Subsystem/2(vbeta)
  Subsystem/1(vdqs) -> vdqs/1

== system Motoring_Gear/alpha-beta//dq3 ==
  valpha_beta : Inport
  *theta_re : Inport  Port=2
  idqs : Inport  Port=3
  Demux : Demux  Outputs=2
  Demux1 : Demux  Outputs=2
  Subsystem : Subsystem
  Subsystem1 : Subsystem
  vdqs : Outport
  ialpha_beta : Outport  Port=2
  wires:
  Subsystem1/1(ialpha_beta) -> ialpha_beta/1
  idqs/1 -> Demux1/1
  valpha_beta/1 -> Demux/1
  *theta_re/1 -> Subsystem1/3(*theta_re1), Subsystem/3(*theta_re)
  Demux1/1 -> Subsystem1/1(id)
  Demux/1 -> Subsystem/1(valpha)
  Demux1/2 -> Subsystem1/2(iq)
  Demux/2 -> Subsystem/2(vbeta)
  Subsystem/1(vdqs) -> vdqs/1

== system Motoring_Gear/alpha-beta//dq4 ==
  valpha_beta : Inport
  *theta_re : Inport  Port=2
  idqs : Inport  Port=3
  Demux : Demux  Outputs=2
  Demux1 : Demux  Outputs=2
  Subsystem : Subsystem
  Subsystem1 : Subsystem
  vdqs : Outport
  ialpha_beta : Outport  Port=2
  wires:
  Subsystem/1(vdqs) -> vdqs/1
  Demux/2 -> Subsystem/2(vbeta)
  Demux1/2 -> Subsystem1/2(iq)
  Demux/1 -> Subsystem/1(valpha)
  Demux1/1 -> Subsystem1/1(id)
  *theta_re/1 -> Subsystem/3(*theta_re), Subsystem1/3(*theta_re1)
  valpha_beta/1 -> Demux/1
  idqs/1 -> Demux1/1
  Subsystem1/1(ialpha_beta) -> ialpha_beta/1

== system Motoring_Gear/power stage1 ==
  iabc : Inport
  Mux1 : Mux  Inputs=3
  Va(10Hz) : Sin  Amplitude=24*sqrt(2/3)  Frequency=2*pi*10  Phase=pi/2  SampleTime=0
  Vb : Sin  Amplitude=24*sqrt(2/3)  Frequency=2*pi*10  Phase=pi/2-2/3*pi  SampleTime=0
  Vc : Sin  Amplitude=24*sqrt(2/3)  Frequency=2*pi*10  Phase=pi/2+2/3*pi  SampleTime=0
  iabc1 : Scope
  vabc1 : Scope
  vabc : Outport
  wires:
  iabc/1 -> iabc1/1
  Vb/1 -> Mux1/2
  Va(10Hz)/1 -> Mux1/1
  Vc/1 -> Mux1/3
  Mux1/1 -> vabc/1, vabc1/1

== system Motoring_Gear/power stage2 ==
  iab : Inport
  Mux1 : Mux  Inputs=2
  Valpha(10Hz) : Sin  Amplitude=24*sqrt(2/3)  Frequency=2*pi*10  Phase=pi/2  SampleTime=0
  Vbeta(10Hz) : Sin  Amplitude=24*sqrt(2/3)  Frequency=2*pi*10  SampleTime=0
  iab1 : Scope
  vab : Scope
  valpha_beta : Outport
  wires:
  Mux1/1 -> vab/1, valpha_beta/1
  iab/1 -> iab1/1
  Valpha(10Hz)/1 -> Mux1/1  "va"
  Vbeta(10Hz)/1 -> Mux1/2  "vb"

== system Motoring_Gear/power stage3 ==
  iabc : Inport
  Mux1 : Mux  Inputs=3
  Mux2 : Mux  Commented=on  Inputs=3
  cos A(10Hz) : Sin  Amplitude=24*sqrt(2/3)  Frequency=0  Phase=pi/2  SampleTime=0
  cos A(10Hz)1 : Sin  Commented=on  Amplitude=24*sqrt(2/3)  Frequency=2*pi*10  Phase=pi/2  SampleTime=0
  cos B : Sin  Amplitude=24*sqrt(2/3)  Frequency=0  Phase=pi/2-2/3*pi  SampleTime=0
  cos B1 : Sin  Commented=on  Amplitude=24*sqrt(2/3)  Frequency=2*pi*10  Phase=pi/2-2/3*pi  SampleTime=0
  cos C : Sin  Amplitude=24*sqrt(2/3)  Frequency=0  Phase=pi/2+2/3*pi  SampleTime=0
  cos C1 : Sin  Commented=on  Amplitude=24*sqrt(2/3)  Frequency=2*pi*10  Phase=pi/2+2/3*pi  SampleTime=0
  iabc1 : Scope
  vabc1 : Scope
  vabc2 : Scope  Commented=on
  vabc : Outport
  wires:
  Mux1/1 -> vabc1/1, vabc/1
  cos C/1 -> Mux1/3
  cos A(10Hz)/1 -> Mux1/1
  cos B/1 -> Mux1/2
  iabc/1 -> iabc1/1
  cos B1/1 -> Mux2/2
  cos A(10Hz)1/1 -> Mux2/1
  cos C1/1 -> Mux2/3
  Mux2/1 -> vabc2/1

== system Motoring_Gear/power stage4 ==
  note: 2*pi*26.57(Wmod fixed)
  note: 2*pi*10
  note: 2*pi*31.55(Wsn fixed)
  iabc : Inport
  Add : Sum  Commented=on
  Mux1 : Mux  Inputs=3
  Tdet : Scope  Commented=on  NumInputPorts=3
  cos A(10Hz) : Sin  Amplitude=24*sqrt(2/3)  Frequency=2*pi*31.55  Phase=pi/2  SampleTime=0
  cos A(10Hz)1 : Sin  Commented=on  Frequency=8*2*pi  SampleTime=0
  cos A(10Hz)2 : Sin  Commented=on  Amplitude=0.08  Frequency=8*4*2*pi  SampleTime=0
  cos B : Sin  Amplitude=24*sqrt(2/3)  Frequency=2*pi*31.55  Phase=pi/2-2/3*pi  SampleTime=0
  cos C : Sin  Amplitude=24*sqrt(2/3)  Frequency=2*pi*31.55  Phase=pi/2+2/3*pi  SampleTime=0
  iabc1 : Scope
  vabc1 : Scope
  vabc : Outport
  wires:
  Mux1/1 -> vabc1/1, vabc/1
  cos C/1 -> Mux1/3
  cos A(10Hz)/1 -> Mux1/1
  cos B/1 -> Mux1/2
  iabc/1 -> iabc1/1
  cos A(10Hz)1/1 -> Tdet/1, Add/1
  cos A(10Hz)2/1 -> Tdet/2, Add/2
  Add/1 -> Tdet/3

== system Motoring_Gear/resolver2 ==
  note: (theta_res_r-theta_res_s)*(-Psn/Pa)=theta_a
  theta_sn,theta_mod : Inport
  Add : Sum  Inputs=-+
  Constant : Constant  Value=2*pi
  Constant1 : Constant  Value=2*pi
  Demux : Demux  Outputs=2
  K_mg : Gain  Gain=-Psn
  Mod : Math  Operator=mod
  Mod1 : Math  Operator=mod
  Mod2 : Math  Operator=mod
  gain : Gain  Gain=q_mod/Psn
  theta_re_res1 : Scope
  theta_res : Scope  NumInputPorts=2
  theta_re_res : Outport
  tag scope: theta_re_res=global
  wires:
  Demux/2 -> gain/1  "theta_mod"
  Demux/1 -> Mod1/1, Add/2  "theta_sn=theta_res_r"
  theta_sn,theta_mod/1 -> Demux/1
  K_mg/1 -> theta_re_res/1, Mod/1
  Add/1 -> K_mg/1  "theta_res_r-theta_res_s"
  gain/1 -> Add/1, Mod2/1  "theta_mod*(qmod/Psn)=theta_res_s"
  Constant/1 -> Mod/2
  Mod1/1 -> theta_res/2
  Constant1/1 -> Mod2/2, Mod1/2
  Mod2/1 -> theta_res/1
  Mod/1 -> theta_re_res1/1, [theta_re_res]

== system Motoring_Gear/Dynamic model1/Subsystem1 ==
  ed : Inport
  eq : Inport  Port=2
  theta_rm : Inport  Port=3
  Add : Sum
  Add1 : Sum
  Cos : Trigonometry  Operator=cos
  Cos1 : Trigonometry
  Cos2 : Trigonometry
  Cos3 : Trigonometry  Operator=cos
  Gain4 : Gain  Gain=-1
  Mux : Mux  Inputs=2
  Product{,1..3} (4 alike) : Product
  ealpha_beta1 : Scope
  edq : Scope  NumInputPorts=2
  ealpha_beta : Outport
  wires:
  Product1/1 -> Add/2
  Add1/1 -> Mux/2
  Cos1/1 -> Gain4/1
  Gain4/1 -> Product1/2
  Cos2/1 -> Product2/2
  Product2/1 -> Add1/1
  Add/1 -> Mux/1
  Product/1 -> Add/1
  Cos3/1 -> Product3/2
  Product3/1 -> Add1/2
  ed/1 -> edq/1, Product/1, Product2/1
  theta_rm/1 -> Cos3/1, Cos2/1, Cos1/1, Cos/1
  Mux/1 -> ealpha_beta1/1, ealpha_beta/1
  eq/1 -> edq/2, Product1/1, Product3/1
  Cos/1 -> Product/2

== system Motoring_Gear/Dynamic model1/Subsystem3 ==
  ealpha_beta : Inport
  Add : Sum  Inputs=-+
  Add1 : Sum  Inputs=--
  Demux1 : Demux  Outputs=2
  Gain1 : Gain  Gain=(1/2)
  Gain2 : Gain  Gain=(1/2)
  Gain3 : Gain  Gain=(sqrt(3)/2)
  Gain6 : Gain  Gain=(sqrt(3)/2)
  Mux1 : Mux  Inputs=3
  ealpha_beta1 : Scope
  eabc : Outport
  wires:
  ealpha_beta/1 -> ealpha_beta1/1, Demux1/1
  Demux1/1 -> Mux1/1, Gain2/1, Gain1/1  "ealpha"
  Mux1/1 -> eabc/1
  Gain1/1 -> Add/1
  Gain6/1 -> Add/2
  Demux1/2 -> Gain3/1, Gain6/1  "ebeta"
  Add/1 -> Mux1/2
  Gain3/1 -> Add1/2
  Gain2/1 -> Add1/1
  Add1/1 -> Mux1/3

== system Motoring_Gear/Load1/DC Motor model(mod) Mod_fixed ==
  note: 聯軸器
  Wmod* : Inport
  Wmod : Inport  Port=2
  Gain1 : Gain  Gain=Kt
  Gain10 : Gain  Gain=Rs_dc
  Gain2 : Gain  Gain=Ke
  Gain3 : Gain  Gain=Kc
  Gain4 : Gain  Gain=1/Ldc
  Gain5 : Gain  Gain=60/(2*pi)
  Gain6 : Gain  Gain=60/(2*pi)
  Integrator : Integrator
  Integrator1 : Integrator
  PI controller : Subsystem
  Sum1 : Sum  Inputs=-+|
  Sum2 : Sum  Inputs=|+-
  Sum4 : Sum  Inputs=-+|
  Sum5 : Sum  Inputs=-+-
  Tmod1 : Scope
  Transfer Fcn1 : TransferFcn  Denominator=[Jdc Bdc]
  wmod : Scope  NumInputPorts=3
  wsn1 : Scope  NumInputPorts=2
  Tmod : Outport
  wires:
  Gain2/1 -> Sum5/3  "e"
  Gain3/1 -> Sum1/1, Tmod1/1, Tmod/1  "Tmod"
  Sum4/1 -> Integrator/1
  Integrator/1 -> Gain3/1
  Wmod/1 -> Sum4/1, Gain5/1, wmod/1
  Transfer Fcn1/1 -> Gain2/1, Gain6/1, Sum2/2, wmod/2, Sum4/2  "Wmod"
  Sum1/1 -> Transfer Fcn1/1
  Gain1/1 -> Sum1/2  "T"
  Sum2/1 -> PI controller/1(error e(t))
  Wmod*/1 -> wmod/3, Sum2/1
  Integrator1/1 -> Gain4/1  "I"
  Sum5/1 -> Integrator1/1
  Gain10/1 -> Sum5/1  "Rs*id"
  PI controller/1(u(t)) -> Sum5/2  "v"
  Gain4/1 -> Gain10/1, Gain1/1
  Gain6/1 -> wsn1/2
  Gain5/1 -> wsn1/1

== system Motoring_Gear/Load1/DC Motor model(sn) ==
  Wsn* : Inport
  Wsn : Inport  Port=2
  Gain1 : Gain  Gain=Kt
  Gain10 : Gain  Gain=Rs_dc
  Gain2 : Gain  Gain=Ke
  Gain3 : Gain  Gain=Kc
  Gain4 : Gain  Gain=1/Ldc
  Gain5 : Gain  Gain=60/(2*pi)
  Gain6 : Gain  Gain=60/(2*pi)
  Integrator : Integrator
  Integrator1 : Integrator
  PI controller : Subsystem
  Sum1 : Sum  Inputs=-+|
  Sum2 : Sum  Inputs=|+-
  Sum4 : Sum  Inputs=-+|
  Sum5 : Sum  Inputs=-+-
  Transfer Fcn1 : TransferFcn  Denominator=[Jdc Bdc]
  Tsn1 : Scope
  v : Scope  NumInputPorts=2
  wsn : Scope  NumInputPorts=3
  wsn1 : Scope  NumInputPorts=2
  Tsn : Outport
  wires:
  Gain10/1 -> Sum5/1  "Rs*id"
  Sum5/1 -> Integrator1/1
  Wsn*/1 -> Sum2/1, wsn/3
  Sum2/1 -> PI controller/1(error e(t))
  PI controller/1(u(t)) -> Sum5/2, v/1  "V"
  Gain1/1 -> Sum1/2  "T"
  Sum1/1 -> Transfer Fcn1/1
  Transfer Fcn1/1 -> Sum4/2, Gain6/1, wsn/2, Sum2/2, Gain2/1  "Wm"
  Wsn/1 -> Gain5/1, wsn/1, Sum4/1
  Integrator/1 -> Gain3/1
  Sum4/1 -> Integrator/1
  Gain3/1 -> Tsn/1, Sum1/1, Tsn1/1  "sn"
  Gain2/1 -> v/2, Sum5/3  "e"
  Integrator1/1 -> Gain4/1  "I"
  Gain4/1 -> Gain10/1, Gain1/1
  Gain5/1 -> wsn1/1
  Gain6/1 -> wsn1/2

== system Motoring_Gear/Load4/DC Motor model(mod) Mod_fixed ==
  note: 聯軸器
  Wmod* : Inport
  Wmod : Inport  Port=2
  Gain1 : Gain  Gain=Kt
  Gain10 : Gain  Gain=Rs_dc
  Gain2 : Gain  Gain=Ke
  Gain3 : Gain  Gain=Kc
  Gain4 : Gain  Gain=1/Ldc
  Integrator : Integrator
  Integrator1 : Integrator
  PI controller : Subsystem
  Sum1 : Sum  Inputs=-+|
  Sum2 : Sum  Inputs=|+-
  Sum4 : Sum  Inputs=-+|
  Sum5 : Sum  Inputs=-+-
  Tmod1 : Scope
  Transfer Fcn1 : TransferFcn  Denominator=[Jdc Bdc]
  wmod : Scope  NumInputPorts=3
  Tmod : Outport
  wires:
  Gain2/1 -> Sum5/3  "e"
  Gain3/1 -> Sum1/1, Tmod1/1, Tmod/1  "Tmod"
  Sum4/1 -> Integrator/1
  Integrator/1 -> Gain3/1
  Wmod/1 -> Sum4/1, wmod/1
  Transfer Fcn1/1 -> Gain2/1, Sum2/2, wmod/2, Sum4/2  "Wmod"
  Sum1/1 -> Transfer Fcn1/1
  Gain1/1 -> Sum1/2  "T"
  Sum2/1 -> PI controller/1(error e(t))
  Wmod*/1 -> wmod/3, Sum2/1
  Integrator1/1 -> Gain4/1  "I"
  Sum5/1 -> Integrator1/1
  Gain10/1 -> Sum5/1  "Rs*id"
  PI controller/1(u(t)) -> Sum5/2  "v"
  Gain4/1 -> Gain10/1, Gain1/1

== system Motoring_Gear/Load4/DC Motor model(sn) ==
  Wsn* : Inport
  Wsn : Inport  Port=2
  Gain1 : Gain  Gain=Kt
  Gain10 : Gain  Gain=Rs_dc
  Gain2 : Gain  Gain=Ke
  Gain3 : Gain  Gain=Kc
  Gain4 : Gain  Gain=1/Ldc
  Integrator : Integrator
  Integrator1 : Integrator
  PI controller : Subsystem
  Sum1 : Sum  Inputs=-+|
  Sum2 : Sum  Inputs=|+-
  Sum4 : Sum  Inputs=-+|
  Sum5 : Sum  Inputs=-+-
  Transfer Fcn1 : TransferFcn  Denominator=[Jdc Bdc]
  Tsn1 : Scope
  v : Scope  NumInputPorts=2
  wsn : Scope  NumInputPorts=3
  Tsn : Outport
  wires:
  Gain10/1 -> Sum5/1  "Rs*id"
  Sum5/1 -> Integrator1/1
  Wsn*/1 -> Sum2/1, wsn/3
  Sum2/1 -> PI controller/1(error e(t))
  PI controller/1(u(t)) -> Sum5/2, v/1  "V"
  Gain1/1 -> Sum1/2  "T"
  Sum1/1 -> Transfer Fcn1/1
  Transfer Fcn1/1 -> Sum4/2, wsn/2, Sum2/2, Gain2/1  "Wm"
  Wsn/1 -> wsn/1, Sum4/1
  Integrator/1 -> Gain3/1
  Sum4/1 -> Integrator/1
  Gain3/1 -> Tsn/1, Sum1/1, Tsn1/1  "Tsn"
  Gain2/1 -> v/2, Sum5/3  "e"
  Integrator1/1 -> Gain4/1  "I"
  Gain4/1 -> Gain10/1, Gain1/1

== system Motoring_Gear/abc//alpha-beta1/Subsystem1 ==
  vabc1 : Inport
  Add : Sum  Inputs=+--
  Add1 : Sum  Inputs=+-
  Demux : Demux  Outputs=3
  Demux1 : Demux  Outputs=3
  Gain : Gain  Gain=2/3
  Gain3 : Gain  Gain=(1/2)
  Gain4 : Gain  Gain=(1/2)
  Gain6 : Gain  Gain=(sqrt(3)/2)
  Gain7 : Gain  Gain=(sqrt(3)/2)
  Mux : Mux  Inputs=2
  valpha_beta2 : Scope
  valpha_beta1 : Outport
  wires:
  Demux1/1 -> ?
  Mux/1 -> valpha_beta1/1, valpha_beta2/1
  Gain3/1 -> Add/2
  Demux/3 -> Gain4/1
  Demux/1 -> Add/1
  Gain4/1 -> Add/3
  vabc1/1 -> Gain/1
  Demux/2 -> Gain3/1
  Add1/1 -> Mux/2
  Demux1/3 -> Gain7/1
  Add/1 -> Mux/1
  Gain/1 -> Demux/1, Demux1/1
  Demux1/2 -> Gain6/1
  Gain6/1 -> Add1/1
  Gain7/1 -> Add1/2

== system Motoring_Gear/abc//alpha-beta1/Subsystem3 ==
  ialpha_beta : Inport
  Add : Sum  Inputs=-+
  Add1 : Sum  Inputs=--
  Demux1 : Demux  Outputs=2
  Gain1 : Gain  Gain=(1/2)
  Gain2 : Gain  Gain=(1/2)
  Gain3 : Gain  Gain=(sqrt(3)/2)
  Gain6 : Gain  Gain=(sqrt(3)/2)
  Mux1 : Mux  Inputs=3
  ialpha_beta1 : Scope
  iabc : Outport
  wires:
  Add1/1 -> Mux1/3
  Gain2/1 -> Add1/1
  Gain3/1 -> Add1/2
  Add/1 -> Mux1/2
  Demux1/2 -> Gain6/1, Gain3/1  "ibeta"
  Gain6/1 -> Add/2
  Gain1/1 -> Add/1
  Mux1/1 -> iabc/1
  Demux1/1 -> Gain1/1, Gain2/1, Mux1/1  "ialpha"
  ialpha_beta/1 -> Demux1/1, ialpha_beta1/1

== system Motoring_Gear/abc//alpha-beta3/Subsystem1 ==
  vabc1 : Inport
  Add : Sum  Inputs=+--
  Add1 : Sum  Inputs=+-
  Demux : Demux  Outputs=3
  Demux1 : Demux  Outputs=3
  Gain : Gain  Gain=2/3
  Gain3 : Gain  Gain=(1/2)
  Gain4 : Gain  Gain=(1/2)
  Gain6 : Gain  Gain=(sqrt(3)/2)
  Gain7 : Gain  Gain=(sqrt(3)/2)
  Mux : Mux  Inputs=2
  valpha_beta2 : Scope
  valpha_beta1 : Outport
  wires:
  Gain7/1 -> Add1/2
  Gain6/1 -> Add1/1
  Demux1/2 -> Gain6/1
  Gain/1 -> Demux1/1, Demux/1
  Add/1 -> Mux/1
  Demux1/3 -> Gain7/1
  Add1/1 -> Mux/2
  Demux/2 -> Gain3/1
  vabc1/1 -> Gain/1
  Gain4/1 -> Add/3
  Demux/1 -> Add/1
  Demux/3 -> Gain4/1
  Gain3/1 -> Add/2
  Mux/1 -> valpha_beta2/1, valpha_beta1/1
  Demux1/1 -> ?

== system Motoring_Gear/abc//alpha-beta3/Subsystem3 ==
  ialpha_beta : Inport
  Add : Sum  Inputs=-+
  Add1 : Sum  Inputs=--
  Demux1 : Demux  Outputs=2
  Gain1 : Gain  Gain=(1/2)
  Gain2 : Gain  Gain=(1/2)
  Gain3 : Gain  Gain=(sqrt(3)/2)
  Gain6 : Gain  Gain=(sqrt(3)/2)
  Mux1 : Mux  Inputs=3
  ialpha_beta1 : Scope
  iabc : Outport
  wires:
  ialpha_beta/1 -> ialpha_beta1/1, Demux1/1
  Demux1/1 -> Mux1/1, Gain2/1, Gain1/1  "ialpha"
  Mux1/1 -> iabc/1
  Gain1/1 -> Add/1
  Gain6/1 -> Add/2
  Demux1/2 -> Gain3/1, Gain6/1  "ibeta"
  Add/1 -> Mux1/2
  Gain3/1 -> Add1/2
  Gain2/1 -> Add1/1
  Add1/1 -> Mux1/3

== system Motoring_Gear/abc//alpha-beta4/Subsystem1 ==
  vabc1 : Inport
  Add : Sum  Inputs=+--
  Add1 : Sum  Inputs=+-
  Demux : Demux  Outputs=3
  Demux1 : Demux  Outputs=3
  Gain : Gain  Gain=2/3
  Gain3 : Gain  Gain=(1/2)
  Gain4 : Gain  Gain=(1/2)
  Gain6 : Gain  Gain=(sqrt(3)/2)
  Gain7 : Gain  Gain=(sqrt(3)/2)
  Mux : Mux  Inputs=2
  valpha_beta2 : Scope
  valpha_beta1 : Outport
  wires:
  Gain7/1 -> Add1/2
  Gain6/1 -> Add1/1
  Demux1/2 -> Gain6/1
  Gain/1 -> Demux1/1, Demux/1
  Add/1 -> Mux/1
  Demux1/3 -> Gain7/1
  Add1/1 -> Mux/2
  Demux/2 -> Gain3/1
  vabc1/1 -> Gain/1
  Gain4/1 -> Add/3
  Demux/1 -> Add/1
  Demux/3 -> Gain4/1
  Gain3/1 -> Add/2
  Mux/1 -> valpha_beta2/1, valpha_beta1/1
  Demux1/1 -> ?

== system Motoring_Gear/abc//alpha-beta4/Subsystem3 ==
  ialpha_beta : Inport
  Add : Sum  Inputs=-+
  Add1 : Sum  Inputs=--
  Demux1 : Demux  Outputs=2
  Gain1 : Gain  Gain=(1/2)
  Gain2 : Gain  Gain=(1/2)
  Gain3 : Gain  Gain=(sqrt(3)/2)
  Gain6 : Gain  Gain=(sqrt(3)/2)
  Mux1 : Mux  Inputs=3
  ialpha_beta1 : Scope
  iabc : Outport
  wires:
  ialpha_beta/1 -> ialpha_beta1/1, Demux1/1
  Demux1/1 -> Mux1/1, Gain2/1, Gain1/1  "ialpha"
  Mux1/1 -> iabc/1
  Gain1/1 -> Add/1
  Gain6/1 -> Add/2
  Demux1/2 -> Gain3/1, Gain6/1  "ibeta"
  Add/1 -> Mux1/2
  Gain3/1 -> Add1/2
  Gain2/1 -> Add1/1
  Add1/1 -> Mux1/3

== system Motoring_Gear/alpha-beta//dq1/Subsystem ==
  valpha : Inport
  vbeta : Inport  Port=2
  *theta_re : Inport  Port=3
  Add : Sum
  Add1 : Sum
  Cos : Trigonometry  Operator=cos
  Cos1 : Trigonometry
  Cos2 : Trigonometry
  Cos3 : Trigonometry  Operator=cos
  Gain3 : Gain  Gain=-1
  Mux : Mux  Inputs=2
  Product{,1..3} (4 alike) : Product
  va_b : Scope  NumInputPorts=2
  vdq : Scope
  vdqs : Outport
  wires:
  Cos/1 -> Product/2
  Product/1 -> Add/1
  Add1/1 -> Mux/2
  Product2/1 -> Add1/1
  Mux/1 -> vdqs/1, vdq/1
  Gain3/1 -> Product2/2
  Product1/1 -> Add/2
  Cos3/1 -> Product3/2
  Cos2/1 -> Gain3/1
  valpha/1 -> Product2/1, Product/1, va_b/1
  Cos1/1 -> Product1/2
  Product3/1 -> Add1/2
  Add/1 -> Mux/1
  vbeta/1 -> Product3/1, Product1/1, va_b/2
  *theta_re/1 -> Cos/1, Cos1/1, Cos2/1, Cos3/1

== system Motoring_Gear/alpha-beta//dq1/Subsystem1 ==
  id : Inport
  iq : Inport  Port=2
  *theta_re1 : Inport  Port=3
  Add : Sum
  Add1 : Sum
  Cos : Trigonometry  Operator=cos
  Cos1 : Trigonometry
  Cos2 : Trigonometry
  Cos3 : Trigonometry  Operator=cos
  Gain4 : Gain  Gain=-1
  Mux : Mux  Inputs=2
  Product{,1..3} (4 alike) : Product
  ialpha_beta1 : Scope
  idq : Scope  NumInputPorts=2
  ialpha_beta : Outport
  wires:
  Cos/1 -> Product/2
  iq/1 -> Product3/1, Product1/1, idq/2
  Mux/1 -> ialpha_beta/1, ialpha_beta1/1
  *theta_re1/1 -> Cos/1, Cos1/1, Cos2/1, Cos3/1
  id/1 -> Product2/1, Product/1, idq/1
  Product3/1 -> Add1/2
  Cos3/1 -> Product3/2
  Product/1 -> Add/1
  Add/1 -> Mux/1
  Product2/1 -> Add1/1
  Cos2/1 -> Product2/2
  Gain4/1 -> Product1/2
  Cos1/1 -> Gain4/1
  Add1/1 -> Mux/2
  Product1/1 -> Add/2

== system Motoring_Gear/alpha-beta//dq2/Subsystem ==
  valpha : Inport
  vbeta : Inport  Port=2
  *theta_re : Inport  Port=3
  Add : Sum
  Add1 : Sum
  Cos : Trigonometry  Operator=cos
  Cos1 : Trigonometry
  Cos2 : Trigonometry
  Cos3 : Trigonometry  Operator=cos
  Gain3 : Gain  Gain=-1
  Mux : Mux  Inputs=2
  Product{,1..3} (4 alike) : Product
  va_b : Scope  NumInputPorts=2
  vdq : Scope
  vdqs : Outport
  wires:
  *theta_re/1 -> Cos3/1, Cos2/1, Cos1/1, Cos/1
  vbeta/1 -> va_b/2, Product1/1, Product3/1
  Add/1 -> Mux/1
  Product3/1 -> Add1/2
  Cos1/1 -> Product1/2
  valpha/1 -> va_b/1, Product/1, Product2/1
  Cos2/1 -> Gain3/1
  Cos3/1 -> Product3/2
  Product1/1 -> Add/2
  Gain3/1 -> Product2/2
  Mux/1 -> vdq/1, vdqs/1
  Product2/1 -> Add1/1
  Add1/1 -> Mux/2
  Product/1 -> Add/1
  Cos/1 -> Product/2

== system Motoring_Gear/alpha-beta//dq2/Subsystem1 ==
  id : Inport
  iq : Inport  Port=2
  *theta_re1 : Inport  Port=3
  Add : Sum
  Add1 : Sum
  Cos : Trigonometry  Operator=cos
  Cos1 : Trigonometry
  Cos2 : Trigonometry
  Cos3 : Trigonometry  Operator=cos
  Gain4 : Gain  Gain=-1
  Mux : Mux  Inputs=2
  Product{,1..3} (4 alike) : Product
  ialpha_beta1 : Scope
  idq : Scope  NumInputPorts=2
  ialpha_beta : Outport
  wires:
  Product1/1 -> Add/2
  Add1/1 -> Mux/2
  Cos1/1 -> Gain4/1
  Gain4/1 -> Product1/2
  Cos2/1 -> Product2/2
  Product2/1 -> Add1/1
  Add/1 -> Mux/1
  Product/1 -> Add/1
  Cos3/1 -> Product3/2
  Product3/1 -> Add1/2
  id/1 -> idq/1, Product/1, Product2/1
  *theta_re1/1 -> Cos3/1, Cos2/1, Cos1/1, Cos/1
  Mux/1 -> ialpha_beta1/1, ialpha_beta/1
  iq/1 -> idq/2, Product1/1, Product3/1
  Cos/1 -> Product/2

== system Motoring_Gear/alpha-beta//dq3/Subsystem ==
  valpha : Inport
  vbeta : Inport  Port=2
  *theta_re : Inport  Port=3
  Add : Sum
  Add1 : Sum
  Cos : Trigonometry  Operator=cos
  Cos1 : Trigonometry
  Cos2 : Trigonometry
  Cos3 : Trigonometry  Operator=cos
  Gain3 : Gain  Gain=-1
  Mux : Mux  Inputs=2
  Product{,1..3} (4 alike) : Product
  va_b : Scope  NumInputPorts=2
  vdq : Scope
  vdqs : Outport
  wires:
  *theta_re/1 -> Cos3/1, Cos2/1, Cos1/1, Cos/1
  vbeta/1 -> va_b/2, Product1/1, Product3/1
  Add/1 -> Mux/1
  Product3/1 -> Add1/2
  Cos1/1 -> Product1/2
  valpha/1 -> va_b/1, Product/1, Product2/1
  Cos2/1 -> Gain3/1
  Cos3/1 -> Product3/2
  Product1/1 -> Add/2
  Gain3/1 -> Product2/2
  Mux/1 -> vdq/1, vdqs/1
  Product2/1 -> Add1/1
  Add1/1 -> Mux/2
  Product/1 -> Add/1
  Cos/1 -> Product/2

== system Motoring_Gear/alpha-beta//dq3/Subsystem1 ==
  id : Inport
  iq : Inport  Port=2
  *theta_re1 : Inport  Port=3
  Add : Sum
  Add1 : Sum
  Cos : Trigonometry  Operator=cos
  Cos1 : Trigonometry
  Cos2 : Trigonometry
  Cos3 : Trigonometry  Operator=cos
  Gain4 : Gain  Gain=-1
  Mux : Mux  Inputs=2
  Product{,1..3} (4 alike) : Product
  ialpha_beta1 : Scope
  idq : Scope  NumInputPorts=2
  ialpha_beta : Outport
  wires:
  Product1/1 -> Add/2
  Add1/1 -> Mux/2
  Cos1/1 -> Gain4/1
  Gain4/1 -> Product1/2
  Cos2/1 -> Product2/2
  Product2/1 -> Add1/1
  Add/1 -> Mux/1
  Product/1 -> Add/1
  Cos3/1 -> Product3/2
  Product3/1 -> Add1/2
  id/1 -> idq/1, Product/1, Product2/1
  *theta_re1/1 -> Cos3/1, Cos2/1, Cos1/1, Cos/1
  Mux/1 -> ialpha_beta1/1, ialpha_beta/1
  iq/1 -> idq/2, Product1/1, Product3/1
  Cos/1 -> Product/2

== system Motoring_Gear/alpha-beta//dq4/Subsystem ==
  valpha : Inport
  vbeta : Inport  Port=2
  *theta_re : Inport  Port=3
  Add : Sum
  Add1 : Sum
  Cos : Trigonometry  Operator=cos
  Cos1 : Trigonometry
  Cos2 : Trigonometry
  Cos3 : Trigonometry  Operator=cos
  Gain3 : Gain  Gain=-1
  Mux : Mux  Inputs=2
  Product{,1..3} (4 alike) : Product
  va_b : Scope  NumInputPorts=2
  vdq : Scope
  vdqs : Outport
  wires:
  Cos/1 -> Product/2
  Product/1 -> Add/1
  Add1/1 -> Mux/2
  Product2/1 -> Add1/1
  Mux/1 -> vdqs/1, vdq/1
  Gain3/1 -> Product2/2
  Product1/1 -> Add/2
  Cos3/1 -> Product3/2
  Cos2/1 -> Gain3/1
  valpha/1 -> Product2/1, Product/1, va_b/1
  Cos1/1 -> Product1/2
  Product3/1 -> Add1/2
  Add/1 -> Mux/1
  vbeta/1 -> Product3/1, Product1/1, va_b/2
  *theta_re/1 -> Cos/1, Cos1/1, Cos2/1, Cos3/1

== system Motoring_Gear/alpha-beta//dq4/Subsystem1 ==
  id : Inport
  iq : Inport  Port=2
  *theta_re1 : Inport  Port=3
  Add : Sum
  Add1 : Sum
  Cos : Trigonometry  Operator=cos
  Cos1 : Trigonometry
  Cos2 : Trigonometry
  Cos3 : Trigonometry  Operator=cos
  Gain4 : Gain  Gain=-1
  Mux : Mux  Inputs=2
  Product{,1..3} (4 alike) : Product
  ialpha_beta1 : Scope
  idq : Scope  NumInputPorts=2
  ialpha_beta : Outport
  wires:
  Cos/1 -> Product/2
  iq/1 -> Product3/1, Product1/1, idq/2
  Mux/1 -> ialpha_beta/1, ialpha_beta1/1
  *theta_re1/1 -> Cos/1, Cos1/1, Cos2/1, Cos3/1
  id/1 -> Product2/1, Product/1, idq/1
  Product3/1 -> Add1/2
  Cos3/1 -> Product3/2
  Product/1 -> Add/1
  Add/1 -> Mux/1
  Product2/1 -> Add1/1
  Cos2/1 -> Product2/2
  Gain4/1 -> Product1/2
  Cos1/1 -> Gain4/1
  Add1/1 -> Mux/2
  Product1/1 -> Add/2

== system Motoring_Gear/Load1/DC Motor model(mod) Mod_fixed/PI controller ==
  error e(t) : Inport
  Add : Sum
  Integrator18 : Integrator
  Ki : Gain  Gain=velocity_Ki_pi+80
  Kp : Gain  Gain=velocity_Kp_pi+25
  u(t) : Outport
  wires:
  error e(t)/1 -> Integrator18/1, Kp/1
  Integrator18/1 -> Ki/1
  Add/1 -> u(t)/1
  Ki/1 -> Add/1
  Kp/1 -> Add/2  "Proportional"

== system Motoring_Gear/Load1/DC Motor model(sn)/PI controller ==
  error e(t) : Inport
  Add : Sum
  Integrator18 : Integrator
  Ki1 : Gain  Gain=velocity_Ki_pi+5
  Kp1 : Gain  Gain=velocity_Kp_pi+10
  u(t) : Outport
  wires:
  Kp1/1 -> Add/2  "Proportional"
  Ki1/1 -> Add/1
  Add/1 -> u(t)/1
  Integrator18/1 -> Ki1/1
  error e(t)/1 -> Kp1/1, Integrator18/1

== system Motoring_Gear/Load4/DC Motor model(mod) Mod_fixed/PI controller ==
  error e(t) : Inport
  Add : Sum
  Integrator18 : Integrator
  Ki : Gain  Gain=velocity_Ki_pi
  Kp : Gain  Gain=velocity_Kp_pi+20
  u(t) : Outport
  wires:
  error e(t)/1 -> Integrator18/1, Kp/1
  Integrator18/1 -> Ki/1
  Add/1 -> u(t)/1
  Ki/1 -> Add/1
  Kp/1 -> Add/2  "Proportional"

== system Motoring_Gear/Load4/DC Motor model(sn)/PI controller ==
  error e(t) : Inport
  Add : Sum
  Integrator18 : Integrator
  Ki1 : Gain  Gain=velocity_Ki_pi+35.5
  Kp1 : Gain  Gain=velocity_Kp_pi+2.1
  u(t) : Outport
  wires:
  Kp1/1 -> Add/2  "Proportional"
  Ki1/1 -> Add/1
  Add/1 -> u(t)/1
  Integrator18/1 -> Ki1/1
  error e(t)/1 -> Kp1/1, Integrator18/1

== matlab function Motoring_Gear/Subsystem2/MATLAB Function23 ==
  data: x input; y output
function y=fcn(x)
if(x>pi)
    y=x-2*pi;
elseif(x<-pi)
    y=x+2*pi;%y=x+2*pi
else
    y=x;
end

== matlab function Motoring_Gear/Subsystem2/MATLAB Function12 ==
  settings: updateMethod=DISCRETE  sampleTime=1e-6
  data: x input; y output
function y=fcn(x)
persistent count old f;
if isempty(count)%初始化
    count = 0;
    f=0;
    old=0;
end

if(f==1 && old-x>3.14 && old>=3.14)%當x變回零時old-x>1.5(2*pi/4) && old>=(2*pi/4)
    count=count+1;
    f=0;
elseif(x>old)    
    f=1;
end
  
y=x+(count*2*pi);%y=x+(count*(2*pi/50))
old=x; 

end
